simulink model "diagrama2"  (Simulink 9.1)
settings: Solver=FixedStepAuto  StartTime=0.0  StopTime=200  FixedStep=0.01  RelTol=1e-3  EnableMultiTasking=on
libraries: commsrccod2 x2, simulink x1
settings Model: Creator=tcom00  LastModifiedBy=erban  ExtModeAutoUpdateStatusClock=off
settings DataIOCC: LimitDataPoints=on  SignalLoggingSaveFormat=ModelDataLogs  SignalLoggingName=sigsOut
settings DebuggingCC: SaveWithParameterizedLinksMsg=none  SignalResolutionControl=TryResolveAllWithWarning  MultiTaskDSMMsg=warning  MultiTaskCondExecSysMsg=none  AllowSymbolicDim=off
settings HardwareCC: TargetUnknown=on

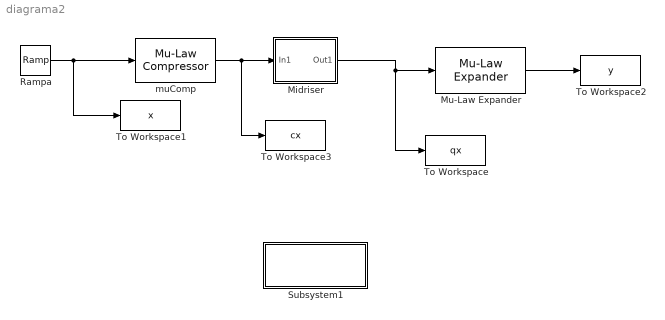
== system diagrama2 ==
  Midriser : Subsystem  mask{L=8, xsc=1}
      mask prompts: L "niveles"
      mask Display: image('.\png\midriser.png');
  Mu-Law Expander : commsrccod2/Mu-Law Expander  mu=10  V=1
      settings: SourceProductName=Communications System Toolbox  SourceProductBaseCode=CM
  Rampa : simulink/Sources/Ramp  slope=0.01  start=0  InitialOutput=-1
  Subsystem1 : Subsystem  mask{mu=10, L=8, xsc=1}
      mask prompts: mu "mu :"; L "Niveles :"; xsc "xsc :"
      mask Callback mu:
      | mu = get_param(gcb, 'mu');
      | set_param([bdroot '/muComp'], 'mu',mu);
      | set_param([bdroot '/Mu-Law Expander'], 'mu',mu);
      mask Callback L:
      | L = get_param(gcb, 'L');
      | set_param([bdroot '/Midriser'], 'L',L);
      mask Callback xsc:
      | xsc = get_param(gcb, 'xsc');
      | set_param([bdroot '/Midriser'], 'xsc',xsc);
      mask Display: disp('Parametros del\nsistema');
  To Workspace : ToWorkspace  VariableName=qx  SampleTime=-1
      settings: Save2DSignal=2-D array (concatenate along first dimension)
  To Workspace1 : ToWorkspace  VariableName=x  SampleTime=-1
      settings: Save2DSignal=2-D array (concatenate along first dimension)
  To Workspace2 : ToWorkspace  VariableName=y  SampleTime=-1
      settings: Save2DSignal=2-D array (concatenate along first dimension)
  To Workspace3 : ToWorkspace  VariableName=cx  SampleTime=-1
      settings: Save2DSignal=2-D array (concatenate along first dimension)
  muComp : commsrccod2/Mu-Law Compressor  mu=10  V=1
      settings: SourceProductName=Communications System Toolbox  SourceProductBaseCode=CM
  wires:
  Rampa/1 -> To Workspace1/1, muComp/1
  muComp/1 -> Midriser/1(In1), To Workspace3/1
  Mu-Law Expander/1 -> To Workspace2/1
  Midriser/1(Out1) -> Mu-Law Expander/1, To Workspace/1

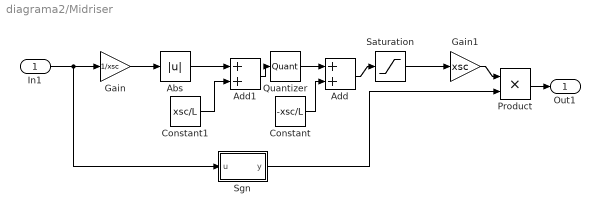
== system diagrama2/Midriser ==
  In1 : Inport
  Abs : Abs
  Add : Sum
  Add1 : Sum
  Constant : Constant  Value=-xsc/L
  Constant1 : Constant  Value=xsc/L
  Gain : Gain  Gain=1/xsc
  Gain1 : Gain  Gain=xsc
  Product : Product
  Quantizer : Quantizer  QuantizationInterval=2*xsc/L
  Saturation : Saturate  UpperLimit=xsc-xsc/L  LowerLimit=-xsc+xsc/L
  Sgn : MATLAB Function  TreatAsAtomicUnit=on
  Out1 : Outport
  wires:
  In1/1 -> Gain/1, Sgn/1(u)
  Product/1 -> Out1/1
  Quantizer/1 -> Add/1
  Sgn/1(y) -> Product/2
  Constant/1 -> Add/2
  Add/1 -> Saturation/1
  Gain1/1 -> Product/1
  Saturation/1 -> Gain1/1
  Add1/1 -> Quantizer/1
  Gain/1 -> Abs/1
  Constant1/1 -> Add1/2
  Abs/1 -> Add1/1

== system diagrama2/Subsystem1 ==

== matlab function Midriser/Sgn ==
  data: u input double; y output double
function y = fcn(u)

if u~=0
    y=sign(u);
else
    y=1;
end
